simulink model "Dc_motor_model_Simscape"  (R2016a)
settings: Solver=VariableStepAuto  StartTime=0.0  StopTime=100  RelTol=1e-3
libraries: fl_lib x9, elec_lib x3, nesl_utility x2
settings Model: Creator=enes_  LastModifiedBy=enes_
settings SimscapeCC: SimscapeLogType=all

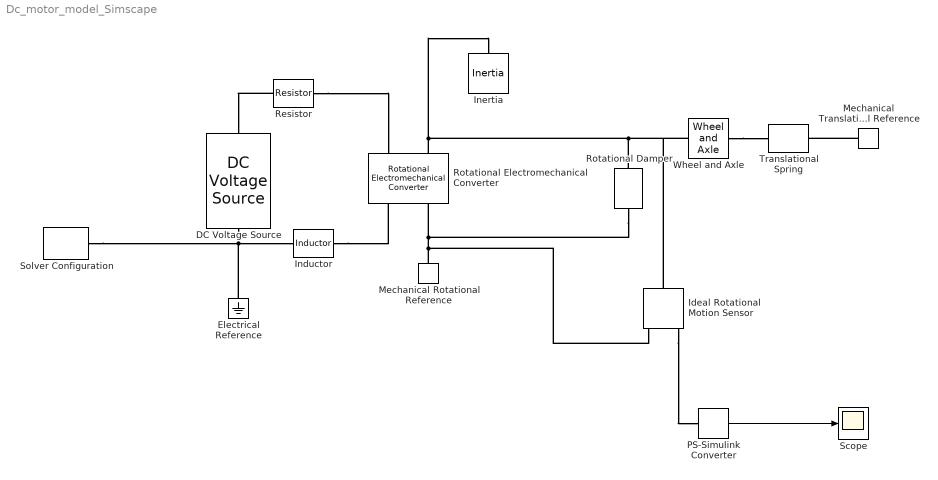
== system Dc_motor_model_Simscape ==
  DC Voltage Source : elec_lib/Additional Components/SPICE-Compatible Components/Sources/DC Voltage Source  DC=220 V
  Electrical Reference : fl_lib/Electrical/Electrical Elements/Electrical Reference
  Ideal Rotational Motion Sensor : fl_lib/Mechanical/Mechanical Sensors/Ideal Rotational Motion Sensor  offset=0 rad
  Inductor : elec_lib/Passive Devices/Inductor  l=1e-6 H  L_tol=20  enable_L_tol=0  tol_distribution=1  nSigma=4  r=0 Ohm  g=1e-9 1/Ohm  initI=0 A  enable_operating_limits=0  operating_limit_action=1  max_working_current=1 A  power_rating=1 W  enable_faults=0  fault_action=1  lambdaPercent=50  k_faulted=0.9999 Ohm  turnsShort=0  openCct=0  groundShort=0  groundShortG=0 1/Ohm  tau_fault=0.001 s  enable_temporal_fault=0  t_fault=1 s  enable_behavioral_fault=0  max_permissible_voltage=100 V  n_fail_on_voltage=1  max_permissible_current=1 A  t_fail_on_current=1 s
  Inertia : fl_lib/Mechanical/Rotational Elements/Inertia  inertia=0.01 kg*m^2  w_specify=off  w_priority=High  w=0 rad/s  t_specify=off  t_priority=None  t=0 N*m
  Mechanical Rotational Reference : fl_lib/Mechanical/Rotational Elements/Mechanical Rotational Reference
  Mechanical Translational Reference : fl_lib/Mechanical/Translational Elements/Mechanical Translational Reference
  PS-Simulink Converter : nesl_utility/PS-Simulink Converter  PhysicalDomain=network_engine_domain  SubClassName=ps_output  LeftPortType=input  RightPortType=output  PseudoPeriodic=off  Frequencies=[]  Unit=1  AffineConversion=off
  Resistor : elec_lib/Passive Devices/Resistor  R=1 Ohm  R_tol=5  enable_R_tol=0  tol_distribution=1  nSigma=4  enable_operating_limits=0  operating_limit_action=2  max_working_voltage=100 V  power_rating=1 W  enable_faults=0  fault_action=1  R_faulted=Inf Ohm  enable_temporal_fault=0  t_fault=1 s  enable_behavioral_fault=0  max_permissible_current=1 A  t_fail_on_current=1 s  noise_mode=0  sample_time=0.001 s  repeatability=1  auto_seed=676943032  user_seed=0  Tdevice=25 degC  alpha=0.00393 1/K  Tmeas=25 degC  thermal_mass=100 J/K  initial_temperature=25 degC  power_derating_T1=70 degC  power_derating_T2=155 degC  operating_temperature_range_vec=[ -50 150 ] degC
  Rotational Electromechanical Converter : fl_lib/Electrical/Electrical Elements/Rotational Electromechanical Converter  K=0.1 V/(rad/s)  i_specify=off  i_priority=None  i=0 A  v_specify=off  v_priority=None  v=0 V  t_specify=off  t_priority=None  t=0 N*m  w_specify=off  w_priority=None  w=0 rad/s
  Rotational Damper : fl_lib/Mechanical/Rotational Elements/Rotational Damper  D=0.001 N*m/(rad/s)  w_specify=off  w_priority=None  w=0 rad/s  t_specify=off  t_priority=None  t=0 N*m
  Scope : Scope
  Solver Configuration : nesl_utility/Solver Configuration  PhysicalDomain=network_engine_domain  SubClassName=solver  LeftPortType=input  RightPortType=generic  Accelerate=off  Tones=[]  Harmonics=[]  SimulateNoise=off  Profile=off  UseLocalSampling=off  EnableSwitchedLinearOptims=on  FrequencyDomain=off  UseCCode=off  RelTol=0.001  AbsTol=1e-06  MinStep=1e-09  ToWorkspace=off  RevertToSquareIcSolve=off  NumHomotopyIterations=100  PhasorMode=off  PhasorModeNumHarmonics=1  OverrideAbsTol=off  DoDC=off  ResidualTolerance=1e-09  UseLocalSolver=off  LocalSolverChoice=NE_BACKWARD_EULER_ADVANCER  LocalSolverSampleTime=0.001  DoFixedCost=off  MaxNonlinIter=3  MaxModeIter=2  LinearAlgebra=Sparse  DelaysMemoryBudget=1024  AutomaticFiltering=on  FilteringTimeConstant=0.001
  Translational Spring : fl_lib/Mechanical/Translational Elements/Translational Spring  spr_rate=1000 N/m  v_specify=off  v_priority=None  v=0 m/s  f_specify=off  f_priority=None  f=0 N  x_specify=off  x_priority=High  x=0 m
  Wheel and Axle : fl_lib/Mechanical/Mechanisms/Wheel and Axle  R=0.05 m  or=1  t_specify=off  t_priority=None  t=0 N*m  f_specify=off  f_priority=None  f=0 N
  wires:
  PS-Simulink Converter/1 -> Scope/1
  connections:
  Resistor/LConn1 -- DC Voltage Source/LConn1
  Resistor/RConn1 -- Rotational Electromechanical Converter/LConn1
  DC Voltage Source/RConn1 -- Solver Configuration/RConn1 -- Electrical Reference/LConn1 -- Inductor/LConn1
  Inductor/RConn1 -- Rotational Electromechanical Converter/RConn1
  Mechanical Rotational Reference/LConn1 -- Ideal Rotational Motion Sensor/RConn1 -- Rotational Damper/RConn1 -- Rotational Electromechanical Converter/RConn2
  Rotational Electromechanical Converter/LConn2 -- Ideal Rotational Motion Sensor/LConn1 -- Wheel and Axle/LConn1 -- Rotational Damper/LConn1 -- Inertia/LConn1
  Wheel and Axle/RConn1 -- Translational Spring/LConn1
  Mechanical Translational Reference/LConn1 -- Translational Spring/RConn1
  Ideal Rotational Motion Sensor/RConn3 -- PS-Simulink Converter/LConn1
